simulink model "sim_all"  (R2020a)
settings: Solver=VariableStepAuto  StartTime=0.0  StopTime=2000  RelTol=1e-3
values from neighbouring files (symbols this model uses):
  a1 = rho * D^4 * alpha1    (= 0.000388302366464)    [data_current.m]
  a2 = -rho * D^3 * alpha2 * (1 - omega)    (= 0.0037030698432)    [data_current.m]
  alpha1 = 0.0113    [data_current.m]
  alpha2 = -0.0091    [data_current.m]
  cornerA = [43.781381 ... (first row only)    [missionC.m]
  cornerB = [43.780975 ... (first row only)    [missionC.m]
  cornerC = [43.780189 ... (first row only)    [missionC.m]
  cornerD = [43.780602 ... (first row only)    [missionC.m]
  ctrl_clockwise = false    [controller.m]
  ctrl_int_bound_or = 0.1    [controller.m]
  ctrl_int_bound_pos = 1    [controller.m]
  ctrl_k_or = 1    [controller.m]
  ctrl_k_pos = 1/3    (= 0.333333333333)    [controller.m]
  ctrl_Ki_vel = 100    [controller.m]
  ctrl_Kp_v_pos = 200    [controller.m]
  ctrl_Kp_vel = 200    [controller.m]
  ctrl_TAM = [  1     1           0           0               0       0;               0     0           1           1               0       0;               0     0           0           0               1       1;               0     0  -(ctrl_r+ctrl_dc)  ctrl_r+ctrl_dc    0       0;               0     0           0           0            -ctrl_r    ctrl_r;           -ctrl_r ctrl_r        0           0       ...(+19 chars)    [controller.m]
  ctrl_Ts = 0.1    [controller.m]
  ctrl_va_uncontrolled = 0.15    [controller.m]
  ctrl_vel_uncontrolled = 0.5    [controller.m]
  D = 0.076    [data_current.m]
  dead_zone_limit = 31.5    [data_current.m]
  depth = 5    [missionC.m]
  distanceFromWall = 8    [missionC.m]
  initInspectedSide = 2    [missionC.m]
  initPoint = [ 43.780796 ... (first row only)    [missionC.m]
  mod_A = pi*mod_R*mod_R    [model.m]
  mod_Cd_F = 0.45    [model.m]
  mod_Cd_M = 0.4    [model.m]
  mod_eta_init = [mod_xNorth; mod_yEast; -mod_zDown; 0; 0; 0]    [model.m]
  mod_g = 9.81    [model.m]
  mod_h0 = 0    [model.m]
  mod_Ixx = mod_Io(1,1)    [model.m]
  mod_Iyy = mod_Io(2,2)    [model.m]
  mod_Izz = mod_Io(3,3)    [model.m]
  mod_Kp_dot = 0    [model.m]
  mod_lat0 = 43.780189    [model.m]
  mod_lon0 = 11.282698    [model.m]
  mod_m = 100    [model.m]
  mod_Mq_dot = mod_Kp_dot    (= 0)    [model.m]
  mod_ni_init = [0; 0; 0; 0; 0; 0]    [model.m]
  mod_Nr_dot = mod_Kp_dot    (= 0)    [model.m]
  mod_p1 = [0; mod_R; 0]    [model.m]
  mod_p2 = [0; -mod_R; 0]    [model.m]
  mod_p3 = [0; 0; (mod_R + mod_z_cm)]    [model.m]
  mod_p4 = [0; 0; -(mod_R + mod_z_cm)]    [model.m]
  mod_p5 = [mod_R; 0; 0]    [model.m]
  mod_p6 = [-mod_R; 0; 0]    [model.m]
  mod_R = ((3*mod_Vol)/(4*pi))^(1/3)    [model.m]
  mod_Rm = (4*mod_R)/(3*pi)    [model.m]
  mod_t1 = [1; 0; 0]    [model.m]
  mod_t2 = [1; 0; 0]    [model.m]
  mod_t3 = [0; 1; 0]    [model.m]
  mod_t4 = [0; 1; 0]    [model.m]
  mod_t5 = [0; 0; 1]    [model.m]
  mod_t6 = [0; 0; 1]    [model.m]
  mod_W = mod_m*mod_g    (= 981)    [model.m]
  mod_Xu_dot = (2/3)*mod_rho_AUV*pi*(mod_R^3)    [model.m]
  mod_Yv_dot = mod_Xu_dot    [model.m]
  mod_z_cm = mod_r_cm(3)    [model.m]
  mod_Zw_dot = mod_Xu_dot    [model.m]
  n_max = 340    [data_current.m]
  nav_DT = 0.1    [navigation.m]
  nav_filter = -1    [data_analysis_simulation_total.m]    (also in navigation.m)
  nav_giro = 2    [navigation.m]
  nav_h0 = 0    [navigation.m]
  nav_lat0 = cornerC(1)    [navigation.m]
  nav_lon0 = cornerC(2)    [navigation.m]
  nav_plane_AB = coefficient_plane(nav_A,nav_B)    [navigation.m]
  nav_plane_BC = coefficient_plane(nav_B,nav_C)    [navigation.m]
  nav_plane_CD = coefficient_plane(nav_C,nav_D)    [navigation.m]
  nav_plane_DA = coefficient_plane(nav_D,nav_A)    [navigation.m]
  nav_resampling = 10000    [navigation.m]
  omega = 0.1    [data_current.m]
  relativeDirection = 30    [missionC.m]
  res_enable_n_eff = 1    [navigation.m]
  rho = 1030    [data_current.m]
  sens_distCM = 0.267    [sensors.m]
  sens_Sample_time_AHRS = 0.1    [sensors.m]
  sens_Sample_time_depth = 0.1    [sensors.m]
  sens_Sample_time_dvl = 0.2    [sensors.m]
  sens_Sample_time_GPS = 1    [sensors.m]
  sens_Sample_time_GYRO = 0.1    [sensors.m]
  sens_Sample_time_sonar = 0.5    [sensors.m]
  sens_threshold = 0.485    [sensors.m]
  sens_Variance_AHRS_pitch = (0.0087)^2    (= 7.569e-05)    [sensors.m]
  sens_Variance_AHRS_roll = (0.0087)^2    (= 7.569e-05)    [sensors.m]
  sens_Variance_AHRS_yaw = (0.0017)^2    (= 2.89e-06)    [sensors.m]
  sens_Variance_depth1 = (0.2)^2    (= 0.04)    [sensors.m]
  sens_Variance_depth2 = (0.4)^2    (= 0.16)    [sensors.m]
  sens_Variance_DVL = (speed*0.03)^2    [sensors.m]
  sens_Variance_GPS = 3    [sensors.m]
  sens_Variance_GYRO = 2.5133e-06    [sensors.m]
  sens_Variance_sonar = 0.05    [sensors.m]
  soglia_or = [0.1, 0.1, 0.1]    [mission.m]
  soglia_orp = 0.1    [mission.m]
  soglia_parete = 0.5    [mission.m]
  soglia_parete_frenata = 0.5    [mission.m]
  soglia_pos = [0.00001, 0.00001, 0.5]    [mission.m]
  soglia_SOS_collisione = 2    [mission.m]
  soglia_SOS_or = [0.25, 0.25, 0.25]    [mission.m]
  soglia_SOS_orp = 0.25    [mission.m]
  soglia_SOS_parete = 1    [mission.m]
  soglia_SOS_pos = [0.00005, 0.00005, 1]    [mission.m]
  soglia_SOS_pos_ris = 2    [mission.m]
  soglia_SOS_vel = 0.2    [mission.m]
  SOS = 0    [mission.m]
  speed = 0.4    [missionC.m]
  stato = 100    [mission.m]
  timer = 40*2    (= 80)    [mission.m]
  Ts_supervisor = 0.1    [mission.m]
undefined symbols (not defined in the file or in its folder): DiscIntNeverNeededParam, nav_A, nav_B, nav_C, nav_D
libraries: simulink x8, cstblocks x6, simulink_extras x1
(part 3 of 8)

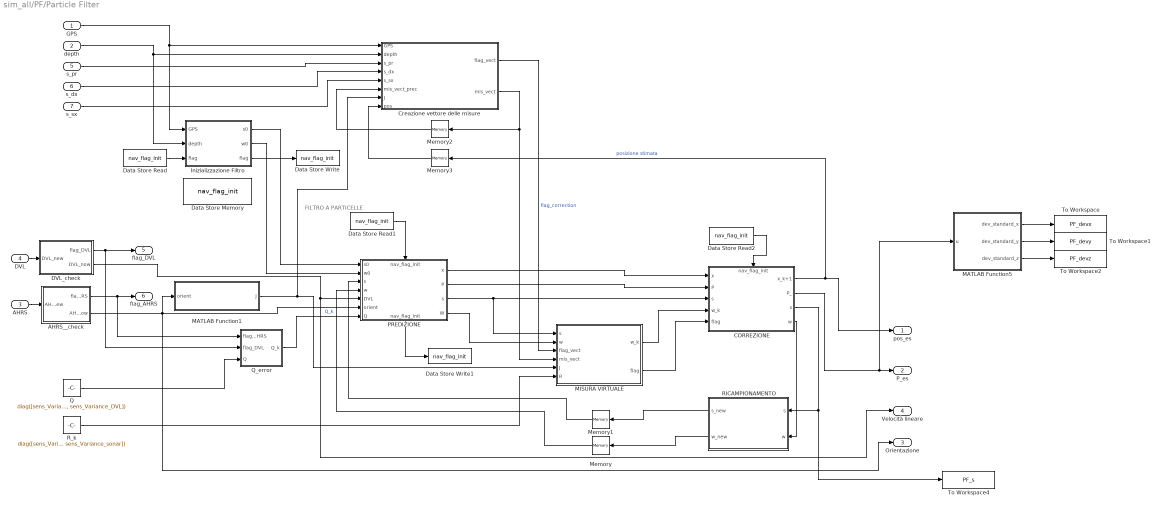
== system sim_all/PF/Particle Filter ==
  note: FILTRO A PARTICELLE
  GPS : Inport
  depth : Inport  Port=2
  AHRS : Inport  Port=3
  DVL : Inport  Port=4
  s_pr : Inport  Port=5
  s_dx : Inport  Port=6
  s_sx : Inport  Port=7
  AHRS__check : Subsystem
  CORREZIONE : Subsystem
      settings: PortSchema="{\"entries\":[{\"content\":{\"sides\":[{\"content\":{\"connectorIds\":[\"In1\",\"In2\",\"In3\",\"In4\",\"In5\"]},\"type\":\"ConnectorPlacement.EquallySpacedRectSide\",\"uuid\":\"067d30f7-0887-4b4f-a6ee-617ba2d59620\"},{\"content\":{\"connectorIds\":[\"Out1\",\"Out2\",\"Out3\",\"Out4\"],\"side\":\"RIGHT\"},\"type\":\"ConnectorPlacement.EquallySpacedRectSide\",\"uuid\":\"6eaec154-fa9b-4277-964e-a31b5cab1928\"},{\"content\":{\"connectorIds\":[\"In6\"],\"side\":\"TOP\"},\"type\":\"ConnectorPlacement.EquallySpacedRectSide\",\"uuid\":\"eb829d42-6933-4b20-85d8-52dfe5077273\"}]},\"type\":\"ConnectorPlacement.EquallySpacedConnector\",\"uuid\":\"d9ec3b67-6d70-427e-aad1-a2dcdcd4b00e\"}],\"packageUris\":[\"http://schema.mathworks.com/mf0/Connector/19700101\"],\"version\":\"1.0\"}"
  Creazione vettore delle misure : MATLAB Function  TreatAsAtomicUnit=on  SystemSampleTime=nav_DT
  DVL_check : Subsystem
  Data Store Memory : DataStoreMemory  DataStoreName=nav_flag_init  ShowAdditionalParam=off
  Data Store Read : DataStoreRead  DataStoreName=nav_flag_init  DataStoreElements=nav_flag_init
  Data Store Read1 : DataStoreRead  DataStoreName=nav_flag_init  DataStoreElements=nav_flag_init
  Data Store Read2 : DataStoreRead  DataStoreName=nav_flag_init  DataStoreElements=nav_flag_init
  Data Store Write : DataStoreWrite  DataStoreName=nav_flag_init  DataStoreElements=nav_flag_init
  Data Store Write1 : DataStoreWrite  DataStoreName=nav_flag_init  DataStoreElements=nav_flag_init
  Inizializzazione Filtro : MATLAB Function  TreatAsAtomicUnit=on  SystemSampleTime=nav_DT
  MATLAB Function1 : MATLAB Function  TreatAsAtomicUnit=on
  MATLAB Function5 : MATLAB Function  TreatAsAtomicUnit=on
  MISURA VIRTUALE : Subsystem
  Memory{,1..3} (4 alike) : Memory
  PREDIZIONE : Subsystem
      settings: PortSchema="{\"entries\":[{\"content\":{\"sides\":[{\"content\":{\"connectorIds\":[\"In1\",\"In2\",\"In3\",\"In4\",\"In5\",\"In6\",\"In7\"]},\"type\":\"ConnectorPlacement.EquallySpacedRectSide\",\"uuid\":\"d45a5da5-05d0-4cdd-84b6-a248ae6e7ceb\"},{\"content\":{\"connectorIds\":[\"Out1\",\"Out2\",\"Out3\",\"Out4\"],\"side\":\"RIGHT\"},\"type\":\"ConnectorPlacement.EquallySpacedRectSide\",\"uuid\":\"47480e48-a9e6-47c5-bf02-88857c9c5826\"},{\"content\":{\"connectorIds\":[\"In8\"],\"side\":\"TOP\"},\"type\":\"ConnectorPlacement.EquallySpacedRectSide\",\"uuid\":\"fce086aa-2512-4880-8bcd-6ad591a282b2\"},{\"content\":{\"connectorIds\":[\"Out5\"],\"side\":\"BOTTOM\"},\"type\":\"ConnectorPlacement.EquallySpacedRectSide\",\"uuid\":\"b6d1202f-9ea1-4bf5-aa1c-3bdf29b80993\"}]},\"type\":\"ConnectorPlacement.EquallySpacedConnector\",\"uuid\":\"773da45d-9f7f-4876-9289-a755558658b5\"}],\"packageUris\":[\"http://schema.mathworks.com/mf0/Connector/19700101\"],\"version\":\"1.0\"}"
  Q : Constant  Value=diag([sens_Variance_AHRS_roll, sens_Variance_AHRS_pitch, sens_Variance_AHRS_yaw, sens_Variance_DVL, sens_Variance_DVL, sens_Variance_DVL])  VectorParams1D=off
  Q_error : Subsystem
  RICAMPIONAMENTO : Subsystem
  R_k : Constant  Value=diag([sens_Variance_GPS, sens_Variance_GPS, sens_Variance_depth1, sens_Variance_sonar, sens_Variance_sonar, sens_Variance_sonar])  VectorParams1D=off
  To Workspace : ToWorkspace  VariableName=PF_devx  SaveFormat=Timeseries  SampleTime=0.1
      settings: Decimation=10
  To Workspace1 : ToWorkspace  VariableName=PF_devy  SaveFormat=Timeseries  SampleTime=0.1
      settings: Decimation=10
  To Workspace2 : ToWorkspace  VariableName=PF_devz  SaveFormat=Timeseries  SampleTime=0.1
      settings: Decimation=10
  To Workspace4 : ToWorkspace  VariableName=PF_s  SaveFormat=Timeseries  SampleTime=0.1
      settings: Decimation=10
  pos_es : Outport  PortDimensions=3
  P_es : Outport  Port=2
  Orientazione : Outport  Port=3
  Velocità lineare : Outport  Port=4
  flag_DVL : Outport  Port=5
  flag_AHRS : Outport  Port=6
  wires:
  Memory/1 -> PREDIZIONE/4(w)
  CORREZIONE/2(P_) -> MATLAB Function5/1(u), P_es/1
  Memory1/1 -> PREDIZIONE/3("s ")
  GPS/1 -> Inizializzazione Filtro/1(GPS), Creazione vettore delle misure/1(GPS)
  depth/1 -> Inizializzazione Filtro/2(depth), Creazione vettore delle misure/2(depth)
  s_pr/1 -> Creazione vettore delle misure/3(s_pr)
  Creazione vettore delle misure/2(mis_vect) -> MISURA VIRTUALE/4(mis_vect), Memory2/1
  Memory2/1 -> Creazione vettore delle misure/6(mis_vect_prec)
  s_dx/1 -> Creazione vettore delle misure/4(s_dx)
  s_sx/1 -> Creazione vettore delle misure/5(s_sx)
  Inizializzazione Filtro/2(w0) -> PREDIZIONE/2(w0)
  Inizializzazione Filtro/1(s0) -> PREDIZIONE/1(s0)
  MATLAB Function1/1(J) -> Creazione vettore delle misure/7(J), MISURA VIRTUALE/5(J)
  Data Store Read/1 -> Inizializzazione Filtro/3("flag ")
  Inizializzazione Filtro/3(flag) -> Data Store Write/1
  Data Store Read1/1 -> PREDIZIONE/8("nav_flag_init ")
  Data Store Read2/1 -> CORREZIONE/6(nav_flag_init)
  PREDIZIONE/5(nav_flag_init) -> Data Store Write1/1
  CORREZIONE/1(x_k+1) -> pos_es/1, Memory3/1  "posizione stimata"
  Memory3/1 -> Creazione vettore delle misure/8(pos)
  AHRS__check/2(AHRS_now) -> PREDIZIONE/6(orient), MATLAB Function1/1(orient), Orientazione/1
  DVL_check/2(DVL_now) -> PREDIZIONE/5(DVL), Velocità lineare/1
  DVL/1 -> DVL_check/1(DVL_new)
  AHRS/1 -> AHRS__check/1(AHRS_new)
  DVL_check/1(flag_DVL) -> flag_DVL/1, Q_error/2(flag_DVL)
  AHRS__check/1(flag_AHRS) -> flag_AHRS/1, Q_error/1(flag_AHRS)
  Q/1 -> Q_error/3(Q)
  Q_error/1(Q_k) -> PREDIZIONE/7(Q)  "Q_k"
  MISURA VIRTUALE/2(flag) -> CORREZIONE/5(flag)
  MISURA VIRTUALE/1(w_k) -> CORREZIONE/4(w_k)
  RICAMPIONAMENTO/1(s_new) -> Memory1/1
  RICAMPIONAMENTO/2(w_new) -> Memory/1
  CORREZIONE/3("s ") -> To Workspace4/1, RICAMPIONAMENTO/1("s ")
  CORREZIONE/4(w) -> RICAMPIONAMENTO/2(w)
  R_k/1 -> MISURA VIRTUALE/6(R)
  Creazione vettore delle misure/1(flag_vect) -> MISURA VIRTUALE/3(flag_vect)  "flag_correction"
  PREDIZIONE/1(x) -> CORREZIONE/1(x)
  PREDIZIONE/2(P) -> CORREZIONE/2(P)
  PREDIZIONE/3(s) -> MISURA VIRTUALE/1(s), CORREZIONE/3(s)
  MATLAB Function5/1(dev_standard_x) -> To Workspace/1
  MATLAB Function5/3(dev_standard_z) -> To Workspace2/1
  MATLAB Function5/2(dev_standard_y) -> To Workspace1/1
  PREDIZIONE/4(W) -> MISURA VIRTUALE/2(w)

== system sim_all/PF/SOS_flag_generator ==
  P_es : Inport
  AHRS : Inport  Port=2
  DVL : Inport  Port=3
  Gyro : Inport  Port=4
  MATLAB Function : MATLAB Function  TreatAsAtomicUnit=on  SystemSampleTime=nav_DT
  Memory : Memory
  nav_SOS : Outport
  tag scope: nav_contatore=global
  wires:
  MATLAB Function/1(SOS) -> nav_SOS/1
  AHRS/1 -> MATLAB Function/3(AHRS)
  DVL/1 -> MATLAB Function/2(DVL)
  P_es/1 -> MATLAB Function/1(P_es)
  [nav_contatore] -> Memory/1
  MATLAB Function/2(contatore) -> [nav_contatore]
  Gyro/1 -> MATLAB Function/4(gyro)
  Memory/1 -> MATLAB Function/5("contatore ")

== system sim_all/Sensors/BLOCCO AHRS1 ==
  note: R  [rad]
      | P  [rad]
  note: Y [rad]
  orient_real : Inport  SampleTime=sens_Sample_time_AHRS
  orient_real1 : Inport  Port=2  SampleTime=sens_Sample_time_AHRS
  orient_real2 : Inport  Port=3  SampleTime=sens_Sample_time_AHRS
  Mux2 : Mux  Inputs=2
  Quantizer : Quantizer  QuantizationInterval=sens_Resolution_AHRS  LinearizeAsGain=off
  Quantizer1 : Quantizer  QuantizationInterval=sens_Resolution_AHRS  LinearizeAsGain=off
  Quantizer2 : Quantizer  QuantizationInterval=sens_Resolution_AHRS  LinearizeAsGain=off
  Random Number : RandomNumber  Variance=sens_Variance_AHRS_roll  Seed=5678  SampleTime=sens_Sample_time_AHRS
  Random Number1 : RandomNumber  Variance=sens_Variance_AHRS_pitch  Seed=4562  SampleTime=sens_Sample_time_AHRS
  Random Number2 : RandomNumber  Variance=sens_Variance_AHRS_yaw  Seed=1258  SampleTime=sens_Sample_time_AHRS
  Sum1 : Sum  Inputs=|++
  Sum2 : Sum  Inputs=++|
  Sum6 : Sum  Inputs=|++
  R-P NED : Outport
  Y NED : Outport  Port=2
  wires:
  orient_real2/1 -> Sum6/1
  orient_real/1 -> Sum2/2
  Sum6/1 -> Quantizer2/1
  Mux2/1 -> R-P NED/1
  Sum2/1 -> Quantizer/1
  orient_real1/1 -> Sum1/1
  Random Number1/1 -> Sum1/2
  Sum1/1 -> Quantizer1/1
  Random Number/1 -> Sum2/1
  Random Number2/1 -> Sum6/2
  Quantizer/1 -> Mux2/1
  Quantizer1/1 -> Mux2/2
  Quantizer2/1 -> Y NED/1

== system sim_all/Sensors/BLOCCO DVL1 ==
  "DVL vx " : Inport  SampleTime=sens_Sample_time_dvl
  DVL vy : Inport  Port=2  SampleTime=sens_Sample_time_dvl
  DVL vz : Inport  Port=3  SampleTime=sens_Sample_time_dvl
  " WNoise DVL x " : RandomNumber  Variance=sens_Variance_DVL  Seed=1234  SampleTime=sens_Sample_time_dvl
  Quantizer : Quantizer  QuantizationInterval=sens_Resolution_dvl  LinearizeAsGain=off
  Quantizer1 : Quantizer  QuantizationInterval=sens_Resolution_dvl  LinearizeAsGain=off
  Quantizer2 : Quantizer  QuantizationInterval=sens_Resolution_dvl  LinearizeAsGain=off
  Sum1 : Sum  Inputs=|++
  Sum2 : Sum  Inputs=|++
  Sum3 : Sum  Inputs=|++
  WNoise DVL y : RandomNumber  Variance=sens_Variance_DVL  Seed=1235  SampleTime=sens_Sample_time_dvl
  WNoise DVL z : RandomNumber  Variance=sens_Variance_DVL  Seed=1237  SampleTime=sens_Sample_time_dvl
  DVL vx BODY : Outport
  DVL vy BODY : Outport  Port=2
  DVL vz BODY : Outport  Port=3
  wires:
  " WNoise DVL x "/1 -> Sum2/2
  Sum2/1 -> Quantizer/1
  WNoise DVL y/1 -> Sum1/2
  Sum1/1 -> Quantizer1/1
  WNoise DVL z/1 -> Sum3/2
  Sum3/1 -> Quantizer2/1
  "DVL vx "/1 -> Sum2/1
  DVL vy/1 -> Sum1/1
  DVL vz/1 -> Sum3/1
  Quantizer/1 -> DVL vx BODY/1
  Quantizer1/1 -> DVL vy BODY/1
  Quantizer2/1 -> DVL vz BODY/1

== system sim_all/Sensors/BLOCCO GPS1 ==
  note: Controllo per antenna
  "LAT " : Inport  SampleTime=sens_Sample_time_GPS
  "LON " : Inport  Port=2  SampleTime=sens_Sample_time_GPS
  DEP : Inport  Port=3  SampleTime=sens_Sample_time_GPS
  Compare To Constant : simulink/Logic and Bit Operations/Compare To Constant  relop=<  const=sens_threshold  OutDataTypeStr=uint8
  Quantizer : Quantizer  QuantizationInterval=sens_Resolution_GPS
  Quantizer1 : Quantizer  QuantizationInterval=sens_Resolution_GPS  LinearizeAsGain=off
  Sum2 : Sum  Inputs=++|
  Sum3 : Sum  Inputs=|++
  WN LAT : RandomNumber  Variance=sens_Variance_GPS  Seed=8765  SampleTime=sens_Sample_time_GPS
  WN LON : RandomNumber  Variance=sens_Variance_GPS  Seed=9876  SampleTime=sens_Sample_time_GPS
  "GPS LAT " : Outport
  "GPS LON " : Outport  Port=2
  FLAG : Outport  Port=3
  wires:
  Sum3/1 -> Quantizer/1
  "LON "/1 -> Sum3/1
  WN LON/1 -> Sum3/2
  Sum2/1 -> Quantizer1/1
  Compare To Constant/1 -> FLAG/1
  DEP/1 -> Compare To Constant/1
  WN LAT/1 -> Sum2/1
  "LAT "/1 -> Sum2/2
  Quantizer1/1 -> "GPS LAT "/1
  Quantizer/1 -> "GPS LON "/1

== system sim_all/Sensors/BLOCCO GYRO1 ==
  angvel_rea1l : Inport  SampleTime=sens_Sample_time_GYRO
  angvel_real2 : Inport  Port=2  SampleTime=sens_Sample_time_GYRO
  angvel_real3 : Inport  Port=3  SampleTime=sens_Sample_time_GYRO
  Clock1 : Clock
  Quantizer : Quantizer  QuantizationInterval=sens_Resolution_GYRO  LinearizeAsGain=off
  Quantizer1 : Quantizer  QuantizationInterval=sens_Resolution_GYRO  LinearizeAsGain=off
  Quantizer2 : Quantizer  QuantizationInterval=sens_Resolution_GYRO  LinearizeAsGain=off
  Subsystem : Subsystem
  Sum1 : Sum  Inputs=+++
  Sum2 : Sum  Inputs=+++
  Sum5 : Sum  Inputs=+++
  WN Gyro P : RandomNumber  Variance=sens_Variance_GYRO  Seed=2347  SampleTime=sens_Sample_time_GYRO
  WN Gyro R : RandomNumber  Variance=sens_Variance_GYRO  Seed=2346  SampleTime=sens_Sample_time_GYRO
  WN Gyro Y : RandomNumber  Variance=sens_Variance_GYRO  Seed=2348  SampleTime=sens_Sample_time_GYRO
  Gyro R BODY : Outport
  Gyro P BODY : Outport  Port=2
  Gyro Y BODY : Outport  Port=3
  wires:
  Sum5/1 -> Quantizer/1
  Sum1/1 -> Quantizer1/1
  Sum2/1 -> Quantizer2/1
  Quantizer/1 -> Gyro R BODY/1
  Quantizer1/1 -> Gyro P BODY/1
  Quantizer2/1 -> Gyro Y BODY/1
  angvel_rea1l/1 -> Sum5/2
  angvel_real2/1 -> Sum1/2
  WN Gyro P/1 -> Sum1/3
  angvel_real3/1 -> Sum2/2
  WN Gyro Y/1 -> Sum2/3
  Clock1/1 -> Subsystem/1(t)
  Subsystem/1(Bias_G) -> Sum2/1, Sum1/1, Sum5/1
  WN Gyro R/1 -> Sum5/3

== system sim_all/Sensors/BLOCCO PROF.1 ==
  note: [m]
  DEP : Inport  SampleTime=sens_Sample_time_depth
  Compare To Constant1 : simulink/Logic and Bit Operations/Compare To Constant  relop=<  const=50  OutDataTypeStr=boolean
  Quantizer : Quantizer  QuantizationInterval=sens_Resolution_depth  LinearizeAsGain=off
  Sum3 : Sum  Inputs=++|
  Switch : Switch  Criteria=u2 > Threshold
  "WN Prof. h< 50 " : RandomNumber  Variance=sens_Variance_depth1  Seed=6543  SampleTime=sens_Sample_time_depth
  WN Prof. h>50 : RandomNumber  Variance=sens_Variance_depth2  Seed=3210  SampleTime=sens_Sample_time_depth
  Profondimetro : Outport
  wires:
  DEP/1 -> Sum3/2, Compare To Constant1/1
  Compare To Constant1/1 -> Switch/2
  "WN Prof. h< 50 "/1 -> Switch/1
  WN Prof. h>50/1 -> Switch/3
  Switch/1 -> Sum3/1
  Sum3/1 -> Quantizer/1
  Quantizer/1 -> Profondimetro/1

== system sim_all/Sensors/Environment and Sensors Model3 ==
  LAT-LON : Inport  SampleTime=sens_Sample_time_sonar
  Environment : Inport  Port=2  SampleTime=sens_Sample_time_sonar
  AHRS Roll : Inport  Port=3  SampleTime=sens_Sample_time_sonar
  AHRS Pitch : Inport  Port=4  SampleTime=sens_Sample_time_sonar
  AHRS Yaw : Inport  Port=5  SampleTime=sens_Sample_time_sonar
  " WN Sonar DX " : RandomNumber  Variance=sens_Variance_sonar  Seed=4325  SampleTime=sens_Sample_time_sonar
  Constant : Constant  Value=sens_distCM
  Demux3 : Demux  Outputs=5
  MATLAB Function1 : MATLAB Function  TreatAsAtomicUnit=on
  Quantizer : Quantizer  QuantizationInterval=sens_Resolution_sonar  LinearizeAsGain=off
  Sum1 : Sum  Inputs=|+-
  Sum2 : Sum  Inputs=|++
  Sonar DX : Outport
  wires:
  MATLAB Function1/1(dist) -> Sum1/1
  Sum1/1 -> Sum2/1
  Constant/1 -> Sum1/2
  Environment/1 -> Demux3/1
  Quantizer/1 -> Sonar DX/1
  Demux3/4 -> MATLAB Function1/5(plane_DA)
  Demux3/2 -> MATLAB Function1/3(plane_BC)
  Sum2/1 -> Quantizer/1
  Demux3/3 -> MATLAB Function1/4(plane_CD)
  AHRS Pitch/1 -> MATLAB Function1/8(Pitch)
  Demux3/1 -> MATLAB Function1/2(plane_AB)
  AHRS Roll/1 -> MATLAB Function1/7(Roll)
  AHRS Yaw/1 -> MATLAB Function1/9(Yaw)
  " WN Sonar DX "/1 -> Sum2/2
  LAT-LON/1 -> MATLAB Function1/1(pos)
  Demux3/5 -> MATLAB Function1/6(plane_W)

== system sim_all/Sensors/Environment and Sensors Model4 ==
  LAT-LON : Inport  SampleTime=sens_Sample_time_sonar
  Environment : Inport  Port=2  SampleTime=sens_Sample_time_sonar
  AHRS Roll : Inport  Port=3  SampleTime=sens_Sample_time_sonar
  AHRS Pitch : Inport  Port=4  SampleTime=sens_Sample_time_sonar
  AHRS Yaw : Inport  Port=5  SampleTime=sens_Sample_time_sonar
  " WN Sonar SX " : RandomNumber  Variance=sens_Variance_sonar  Seed=4321  SampleTime=sens_Sample_time_sonar
  Constant : Constant  Value=sens_distCM
  Demux3 : Demux  Outputs=5
  MATLAB Function1 : MATLAB Function  TreatAsAtomicUnit=on
  Quantizer : Quantizer  QuantizationInterval=sens_Resolution_sonar  LinearizeAsGain=off
  Sum1 : Sum  Inputs=|+-
  Sum2 : Sum  Inputs=|++
  Sonar SX : Outport
  wires:
  MATLAB Function1/1(dist) -> Sum1/1
  Sum1/1 -> Sum2/1
  Constant/1 -> Sum1/2
  Environment/1 -> Demux3/1
  Quantizer/1 -> Sonar SX/1
  Demux3/4 -> MATLAB Function1/5(plane_DA)
  Demux3/2 -> MATLAB Function1/3(plane_BC)
  Sum2/1 -> Quantizer/1
  Demux3/3 -> MATLAB Function1/4(plane_CD)
  AHRS Pitch/1 -> MATLAB Function1/8(Pitch)
  Demux3/1 -> MATLAB Function1/2(plane_AB)
  AHRS Roll/1 -> MATLAB Function1/7(Roll)
  AHRS Yaw/1 -> MATLAB Function1/9(Yaw)
  " WN Sonar SX "/1 -> Sum2/2
  LAT-LON/1 -> MATLAB Function1/1(pos)
  Demux3/5 -> MATLAB Function1/6(plane_W)

== system sim_all/Sensors/Environment and Sensors Model6 ==
  LAT-LON : Inport  SampleTime=sens_Sample_time_sonar
  Environment : Inport  Port=2  SampleTime=sens_Sample_time_sonar
  AHRS Roll : Inport  Port=3  SampleTime=sens_Sample_time_sonar
  AHRS Pitch : Inport  Port=4  SampleTime=sens_Sample_time_sonar
  AHRS Yaw : Inport  Port=5  SampleTime=sens_Sample_time_sonar
  " WN Sonar Prua " : RandomNumber  Variance=sens_Variance_sonar  Seed=1234  SampleTime=sens_Sample_time_sonar
  Constant : Constant  Value=sens_distCM
  Demux3 : Demux  Outputs=5
  MATLAB Function1 : MATLAB Function  TreatAsAtomicUnit=on
  Quantizer : Quantizer  QuantizationInterval=sens_Resolution_sonar  LinearizeAsGain=off
  Sum1 : Sum  Inputs=|+-
  Sum2 : Sum  Inputs=|++
  Sonar Prua : Outport
  wires:
  Demux3/3 -> MATLAB Function1/4(plane_CD)
  " WN Sonar Prua "/1 -> Sum2/2
  LAT-LON/1 -> MATLAB Function1/1(pos)
  Demux3/1 -> MATLAB Function1/2(plane_AB)
  Demux3/4 -> MATLAB Function1/5(plane_DA)
  Sum2/1 -> Quantizer/1
  Demux3/2 -> MATLAB Function1/3(plane_BC)
  Quantizer/1 -> Sonar Prua/1
  Environment/1 -> Demux3/1
  AHRS Roll/1 -> MATLAB Function1/7(Roll)
  AHRS Pitch/1 -> MATLAB Function1/8(Pitch)
  AHRS Yaw/1 -> MATLAB Function1/9(Yaw)
  MATLAB Function1/1(dist) -> Sum1/1
  Sum1/1 -> Sum2/1
  Constant/1 -> Sum1/2
  Demux3/5 -> MATLAB Function1/6(plane_W)

== system sim_all/Controller_mk4_v3/C_or/C_va_X_td ==
  err_va : Inport
  Reset : ResetPort  DisableCoverage=on
  LTI System : cstblocks/LTI System  sys=ctrl_Cva_td3  IC=[]
  tau : Outport
  wires:
  err_va/1 -> LTI System/1
  LTI System/1 -> tau/1

== system sim_all/Controller_mk4_v3/C_or/C_va_Y_td ==
  err_va : Inport
  Reset : ResetPort  DisableCoverage=on
  LTI System : cstblocks/LTI System  sys=ctrl_Cva_td3  IC=[]
  tau : Outport
  wires:
  LTI System/1 -> tau/1
  err_va/1 -> LTI System/1

== system sim_all/Controller_mk4_v3/C_or/C_va_Z_td ==
  err_va : Inport
  Reset : ResetPort  DisableCoverage=on
  LTI System : cstblocks/LTI System  sys=ctrl_Cva_td3  IC=[]
  tau : Outport
  wires:
  err_va/1 -> LTI System/1
  LTI System/1 -> tau/1

== system sim_all/Controller_mk4_v3/C_pos/abs_integrator1 ==
  err_x : Inport
  err_y : Inport  Port=2
  err_z : Inport  Port=3
  enabler : Inport  Port=4
  Body2Ned : MATLAB Function  TreatAsAtomicUnit=on
  Demux : Demux  Outputs=3
  Discrete-Time Integrator : DiscreteIntegrator  gainval=ctrl_Ki_pos  ExternalReset=rising  SampleTime=ctrl_Ts  ICPrevOutput=DiscIntNeverNeededParam  ICPrevScaledInput=DiscIntNeverNeededParam
  Mux : Mux  Inputs=3
  Ned2Body1 : MATLAB Function  TreatAsAtomicUnit=on
  int_x : Outport
  int_y : Outport  Port=2
  int_z : Outport  Port=3
  wires:
  [Or] -> Ned2Body1/2(or), Body2Ned/2(or)
  enabler/1 -> Discrete-Time Integrator/2
  Body2Ned/1(x_n) -> Discrete-Time Integrator/1
  err_x/1 -> Mux/1
  err_y/1 -> Mux/2
  Mux/1 -> Body2Ned/1(x_b)
  Ned2Body1/1(x_b) -> Demux/1
  Demux/1 -> int_x/1
  Demux/2 -> int_y/1
  Demux/3 -> int_z/1
  err_z/1 -> Mux/3
  Discrete-Time Integrator/1 -> Ned2Body1/1(x_n)

== system sim_all/Controller_mk4_v3/C_pos/abs_integrator2 ==
  err_vx : Inport
  err_vy : Inport  Port=2
  err_vz : Inport  Port=3
  enabler : Inport  Port=4
  Body2Ned : MATLAB Function  TreatAsAtomicUnit=on
  Demux : Demux  Outputs=3
  Discrete-Time Integrator : DiscreteIntegrator  gainval=ctrl_Ki_v_pos  ExternalReset=rising  SampleTime=ctrl_Ts  ICPrevOutput=DiscIntNeverNeededParam  ICPrevScaledInput=DiscIntNeverNeededParam
  Mux : Mux  Inputs=3
  Ned2Body1 : MATLAB Function  TreatAsAtomicUnit=on
  int_vx : Outport
  int_vy : Outport  Port=2
  int_vz : Outport  Port=3
  wires:
  Demux/3 -> int_vz/1
  Demux/2 -> int_vy/1
  Demux/1 -> int_vx/1
  Ned2Body1/1(x_b) -> Demux/1
  Mux/1 -> Body2Ned/1(x_b)
  err_vy/1 -> Mux/2
  err_vx/1 -> Mux/1
  [Or] -> Body2Ned/2(or), Ned2Body1/2(or)
  err_vz/1 -> Mux/3
  Body2Ned/1(x_n) -> Discrete-Time Integrator/1
  enabler/1 -> Discrete-Time Integrator/2
  Discrete-Time Integrator/1 -> Ned2Body1/1(x_n)

== system sim_all/Controller_mk4_v3/C_vel/abs_integrator ==
  err_vx : Inport
  err_vy : Inport  Port=2
  err_vz : Inport  Port=3
  enabler : Inport  Port=4
  Body2Ned : MATLAB Function  TreatAsAtomicUnit=on
  Demux : Demux  Outputs=3
  Discrete-Time Integrator : DiscreteIntegrator  gainval=ctrl_Ki_vel  ExternalReset=rising  SampleTime=ctrl_Ts  ICPrevOutput=DiscIntNeverNeededParam  ICPrevScaledInput=DiscIntNeverNeededParam
  Mux : Mux  Inputs=3
  Ned2Body1 : MATLAB Function  TreatAsAtomicUnit=on
  int_vx : Outport
  int_vy : Outport  Port=2
  int_vz : Outport  Port=3
  wires:
  Demux/3 -> int_vz/1
  Demux/2 -> int_vy/1
  Demux/1 -> int_vx/1
  Ned2Body1/1(x_b) -> Demux/1
  Mux/1 -> Body2Ned/1(x_b)
  err_vy/1 -> Mux/2
  err_vx/1 -> Mux/1
  [Or] -> Body2Ned/2(or), Ned2Body1/2(or)
  err_vz/1 -> Mux/3
  Body2Ned/1(x_n) -> Discrete-Time Integrator/1
  enabler/1 -> Discrete-Time Integrator/2
  Discrete-Time Integrator/1 -> Ned2Body1/1(x_n)

== system sim_all/Controller_mk4_v3/signal_to_NED/Signal_d->NED ==
  Vel_d : Inport
  Dpp_d : Inport  Port=2
  Dps_d : Inport  Port=3
  Orp_d : Inport  Port=4
  Wall : Inport  Port=5
  ToNed : MATLAB Function  TreatAsAtomicUnit=on
  wall_fcn : MATLAB Function  TreatAsAtomicUnit=on
  Vel_d_ned : Outport  VectorParamsAs1DForOutWhenUnconnected=off
  Dpp_d_ned : Outport  Port=2  VectorParamsAs1DForOutWhenUnconnected=off
  Dps_d_ned : Outport  Port=3  VectorParamsAs1DForOutWhenUnconnected=off
  Orp_d_ned : Outport  Port=4  VectorParamsAs1DForOutWhenUnconnected=off
  wires:
  wall_fcn/1(wall_vect) -> ToNed/5(wall_vect)
  ToNed/3(dps_n) -> Dps_d_ned/1
  Wall/1 -> wall_fcn/1(WALL)
  Dpp_d/1 -> ToNed/2(ddp)
  ToNed/2(ddp_n) -> Dpp_d_ned/1
  ToNed/1(vel_n) -> Vel_d_ned/1
  Orp_d/1 -> ToNed/4(orp)
  ToNed/4(orp_n) -> Orp_d_ned/1
  Dps_d/1 -> ToNed/3(dps)
  Vel_d/1 -> ToNed/1(vel)
  wall_fcn/2(wall_vect2) -> ToNed/6(wall_vect2)
  [current_state] -> ToNed/7(state)

== system sim_all/Controller_mk4_v3/signal_to_NED/Signal_s->NED ==
  Dpp_s : Inport
  Dps_s : Inport  Port=2
  Wall : Inport  Port=3
  ToNed : MATLAB Function  TreatAsAtomicUnit=on
  wall_fcn1 : MATLAB Function  TreatAsAtomicUnit=on
  Dpp_s_ned : Outport  VectorParamsAs1DForOutWhenUnconnected=off
  Dps_s_ned : Outport  Port=2  VectorParamsAs1DForOutWhenUnconnected=off
  wires:
  Dpp_s/1 -> ToNed/1(ddp)
  ToNed/1(ddp_n) -> Dpp_s_ned/1
  Dps_s/1 -> ToNed/2(dps)
  ToNed/2(dps_n) -> Dps_s_ned/1
  Wall/1 -> wall_fcn1/1(WALL)
  wall_fcn1/1(wall_vect) -> ToNed/3(wall_vect)
  wall_fcn1/2(wall_vect2) -> ToNed/4(wall_vect2)

== system sim_all/EKF/Extended Kalman Filter/AHRS__check ==
  AHRS_new : Inport
  MATLAB Function4 : MATLAB Function  TreatAsAtomicUnit=on
  Memory4 : Memory
  flag_AHRS : Outport
  AHRS_now : Outport  Port=2
  wires:
  AHRS_new/1 -> MATLAB Function4/1(AHRS_new)
  Memory4/1 -> MATLAB Function4/2(AHRS_old)
  MATLAB Function4/1(flag_AHRS) -> flag_AHRS/1
  MATLAB Function4/2(AHRS_now) -> Memory4/1, AHRS_now/1

== system sim_all/EKF/Extended Kalman Filter/CORREZIONE ==
  x_k|k-1 : Inport
  P_k|k-1 : Inport  Port=2
  e : Inport  Port=3
  H : Inport  Port=4
  R : Inport  Port=5
  nav_flag_init : Inport  Port=6
  MATLAB Function : MATLAB Function  TreatAsAtomicUnit=on  SystemSampleTime=nav_DT
  x_k|k : Outport
  P_k|k : Outport  Port=2
  wires:
  x_k|k-1/1 -> MATLAB Function/1(x_k_k_1)
  P_k|k-1/1 -> MATLAB Function/2(P_k_k_1)
  e/1 -> MATLAB Function/3(e)
  H/1 -> MATLAB Function/4(H)
  MATLAB Function/1(x_k) -> x_k|k/1
  MATLAB Function/2(P_k) -> P_k|k/1
  nav_flag_init/1 -> MATLAB Function/6(nav_flag_init)
  R/1 -> MATLAB Function/5(R_k)

== system sim_all/EKF/Extended Kalman Filter/DVL_check ==
  DVL_new : Inport
  MATLAB Function4 : MATLAB Function  TreatAsAtomicUnit=on
  Memory4 : Memory
  flag_DVL : Outport
  DVL_now : Outport  Port=2
  wires:
  DVL_new/1 -> MATLAB Function4/1(DVL_new)
  Memory4/1 -> MATLAB Function4/2(DVL_old)
  MATLAB Function4/1(flag_DVL) -> flag_DVL/1
  MATLAB Function4/2(DVL_now) -> Memory4/1, DVL_now/1

== system sim_all/EKF/Extended Kalman Filter/MISURA VIRTUALE ==
  x_k|k-1 : Inport
  flag_vect : Inport  Port=2
  mis_vect : Inport  Port=3
  J : Inport  Port=4
  MATLAB Function : MATLAB Function  TreatAsAtomicUnit=on  SystemSampleTime=nav_DT
  e : Outport
  H : Outport  Port=2
  wires:
  x_k|k-1/1 -> MATLAB Function/1(x_k_k_1)
  mis_vect/1 -> MATLAB Function/3(mis_vect)
  flag_vect/1 -> MATLAB Function/2(flag_vect)
  MATLAB Function/1(e) -> e/1
  MATLAB Function/2(H) -> H/1
  J/1 -> MATLAB Function/4(J)

== system sim_all/EKF/Extended Kalman Filter/PREDIZIONE ==
  x0 : Inport
  P0 : Inport  Port=2
  x_k-1|k-1 : Inport  Port=3
  u_k-1 : Inport  Port=4
  P_k-1|k-1 : Inport  Port=5
  J : Inport  Port=6
  L : Inport  Port=7
  Q_k-1 : Inport  Port=8
  nav_flag_init : Inport  Port=9
  Passo di Predizione : MATLAB Function  TreatAsAtomicUnit=on  SystemSampleTime=nav_DT
  x_k|k-1 : Outport
  P_k|k-1 : Outport  Port=2
  flag_init : Outport  Port=3
  wires:
  Passo di Predizione/1(x_k) -> x_k|k-1/1
  Passo di Predizione/2(P_k) -> P_k|k-1/1
  u_k-1/1 -> Passo di Predizione/4(u_k_1)
  x_k-1|k-1/1 -> Passo di Predizione/3(x_k_1)
  P_k-1|k-1/1 -> Passo di Predizione/5(P_k_1)
  J/1 -> Passo di Predizione/6(J)
  Q_k-1/1 -> Passo di Predizione/8(Q_k_1)
  P0/1 -> Passo di Predizione/2(P0)
  x0/1 -> Passo di Predizione/1(x0)
  L/1 -> Passo di Predizione/7(L)
  nav_flag_init/1 -> Passo di Predizione/9("nav_flag_init ")
  Passo di Predizione/3(nav_flag_init) -> flag_init/1

== system sim_all/EKF/Extended Kalman Filter/Q_error ==
  flag_AHRS : Inport
  flag_DVL : Inport  Port=2
  Q : Inport  Port=3
  MATLAB Function4 : MATLAB Function  TreatAsAtomicUnit=on
  Memory : Memory
  Q_k : Outport
  wires:
  MATLAB Function4/1(Q_k) -> Q_k/1, Memory/1
  flag_AHRS/1 -> MATLAB Function4/3(flag_AHRS)
  flag_DVL/1 -> MATLAB Function4/4(flag_DVL)
  Memory/1 -> MATLAB Function4/2(Q_k_1)
  Q/1 -> MATLAB Function4/1(Q)

== system sim_all/Mission_supervisor_v3/Mission_Supervisor/Completamento ==
  parete : Inport
  Pos_s : Inport  Port=2
  Vel_s : Inport  Port=3
  Dpp_s : Inport  Port=4
  Dps_s : Inport  Port=5
  Orp_s : Inport  Port=6
  Dps_fin : Inport  Port=7
  error_flag : Inport  Port=8
  giro : Inport  Port=9
  Action Port : ActionPort  ActionPortLabel=case [ 204 ]:
  Constant{,1..2,6} (4 alike) : Constant  Value=nan
  MATLAB Function : MATLAB Function  TreatAsAtomicUnit=on  SystemSampleTime=Ts_supervisor
  Mux : Mux  Inputs=6
  Mux1 : Mux  Inputs=3
  delta_current_comp : Outport
  delta_stato_comp : Outport  Port=2
  Outport : Outport  Port=3
  wires:
  MATLAB Function/1(delta_current_comp) -> delta_current_comp/1
  MATLAB Function/2(delta_stato_comp) -> delta_stato_comp/1
  parete/1 -> MATLAB Function/1(parete)
  MATLAB Function/3(Pos_d) -> Mux/1
  Mux/1 -> Outport/1
  MATLAB Function/4(Vel_d) -> Mux/3
  MATLAB Function/5(Dpp_d) -> Mux/4
  MATLAB Function/6(Orp_d) -> Mux/6
  Constant/1 -> Mux1/1
  Constant1/1 -> Mux1/2
  Constant6/1 -> Mux1/3
  Mux1/1 -> Mux/2
  Constant2/1 -> Mux/5
  Pos_s/1 -> MATLAB Function/2(Pos_s)
  Vel_s/1 -> MATLAB Function/3(Vel_s)
  Dpp_s/1 -> MATLAB Function/4(Dpp_s)
  Dps_s/1 -> MATLAB Function/5(Dps_s)
  Orp_s/1 -> MATLAB Function/6(Orp_s)
  Dps_fin/1 -> MATLAB Function/7(dps_fin)
  error_flag/1 -> MATLAB Function/8(error_flag)
  giro/1 -> MATLAB Function/9(giro)

== system sim_all/Mission_supervisor_v3/Mission_Supervisor/Fine missione ==
  current_state : Inport
  Action Port : ActionPort  ActionPortLabel=case [ 304 ]:
  Constant{1..7} (7 alike) : Constant  Value=nan
  MATLAB Function : MATLAB Function  TreatAsAtomicUnit=on  SystemSampleTime=Ts_supervisor
  Mux : Mux  Inputs=6
  Mux1 : Mux  Inputs=3
  delta_current_end : Outport
  Outport : Outport  Port=2
  wires:
  MATLAB Function/1(delta_current_end) -> delta_current_end/1
  current_state/1 -> MATLAB Function/1(stato)
  Mux/1 -> Outport/1
  Constant2/1 -> Mux/3
  Constant3/1 -> Mux/4
  Constant4/1 -> Mux/5
  Constant5/1 -> Mux/6
  Constant1/1 -> Mux1/1
  Constant6/1 -> Mux1/2
  Constant7/1 -> Mux1/3
  Mux1/1 -> Mux/1, Mux/2

== system sim_all/Mission_supervisor_v3/Mission_Supervisor/Frenata in completamento ==
  Pos_s : Inport
  Orp_s : Inport  Port=2
  Dpp_s : Inport  Port=3
  Dps_s : Inport  Port=4
  dps_fin : Inport  Port=5
  error_flag : Inport  Port=6
  Action Port : ActionPort  ActionPortLabel=case [ 205 ]:
  Constant{,1..2,6} (4 alike) : Constant  Value=nan
  MATLAB Function : MATLAB Function  TreatAsAtomicUnit=on  SystemSampleTime=Ts_supervisor
  Mux : Mux  Inputs=6
  Mux1 : Mux  Inputs=3
  delta_current_fren_comp : Outport
  delta_stato_fren_comp : Outport  Port=2
  SOS_205 : Outport  Port=3
  " " : Outport  Port=4
  wires:
  MATLAB Function/1(delta_current_fren_comp) -> delta_current_fren_comp/1
  MATLAB Function/2(delta_stato_fren_comp) -> delta_stato_fren_comp/1
  MATLAB Function/4(Pos_d) -> Mux/1
  MATLAB Function/5(Dpp_d) -> Mux/4
  MATLAB Function/6(Dps_d) -> Mux/5
  MATLAB Function/7(Orp_d) -> Mux/6
  Constant/1 -> Mux1/1
  Constant1/1 -> Mux1/2
  Constant6/1 -> Mux1/3
  Mux1/1 -> Mux/2
  Constant2/1 -> Mux/3
  Pos_s/1 -> MATLAB Function/1(Pos_s)
  Orp_s/1 -> MATLAB Function/2(Orp_s)
  Dpp_s/1 -> MATLAB Function/3(Dpp_s)
  Dps_s/1 -> MATLAB Function/4(Dps_s)
  dps_fin/1 -> MATLAB Function/5(dps_fin)
  error_flag/1 -> MATLAB Function/6(error_flag)
  MATLAB Function/3(SOS_205) -> SOS_205/1
  Mux/1 -> " "/1

== system sim_all/Mission_supervisor_v3/Mission_Supervisor/Frenata pattugliamento ==
  contatore : Inport
  Pos_s : Inport  Port=2
  Dpp_s : Inport  Port=3
  Dps_s : Inport  Port=4
  Orp_s : Inport  Port=5
  error_flag : Inport  Port=6
  Action Port : ActionPort  ActionPortLabel=case [ 202 ]:
  Constant{,1..2,6} (4 alike) : Constant  Value=nan
  MATLAB Function : MATLAB Function  TreatAsAtomicUnit=on  SystemSampleTime=Ts_supervisor
  Mux : Mux  Inputs=6
  Mux1 : Mux  Inputs=3
  delta_current_fren_patt : Outport
  delta_stato_fren_patt : Outport  Port=2
  Outport : Outport  Port=3
  wires:
  MATLAB Function/1(delta_current_fren_patt) -> delta_current_fren_patt/1
  MATLAB Function/2(delta_stato_fren_patt) -> delta_stato_fren_patt/1
  MATLAB Function/3(Pos_d) -> Mux/1
  Mux/1 -> Outport/1
  contatore/1 -> MATLAB Function/1(contatore)
  MATLAB Function/4(Dpp_d) -> Mux/4
  MATLAB Function/5(Dps_d) -> Mux/5
  MATLAB Function/6(Orp_d) -> Mux/6
  Constant/1 -> Mux1/1
  Constant1/1 -> Mux1/2
  Constant6/1 -> Mux1/3
  Mux1/1 -> Mux/2
  Constant2/1 -> Mux/3
  Pos_s/1 -> MATLAB Function/2(Pos_s)
  Dpp_s/1 -> MATLAB Function/3(Dpp_s)
  Dps_s/1 -> MATLAB Function/4(Dps_s)
  Orp_s/1 -> MATLAB Function/5(Orp_s)
  error_flag/1 -> MATLAB Function/6(error_flag)

== system sim_all/Mission_supervisor_v3/Mission_Supervisor/Immersione ==
  Pos_s : Inport
  punto_iniz_patt : Inport  Port=2
  Or_in : Inport  Port=3
  error_flag : Inport  Port=4
  Action Port : ActionPort  ActionPortLabel=case [ 103 ]:
  Constant{,1..3} (4 alike) : Constant  Value=nan
  MATLAB Function : MATLAB Function  TreatAsAtomicUnit=on  SystemSampleTime=Ts_supervisor
  Mux : Mux  Inputs=6
  delta_current_immers : Outport
  delta_stato_immers : Outport  Port=2
  Outport : Outport  Port=3
  wires:
  MATLAB Function/1(delta_current_immers) -> delta_current_immers/1
  MATLAB Function/2(delta_stato_immers) -> delta_stato_immers/1
  MATLAB Function/3(Pos_d) -> Mux/1
  Mux/1 -> Outport/1
  Constant/1 -> Mux/3
  Constant1/1 -> Mux/6
  Constant2/1 -> Mux/5
  Pos_s/1 -> MATLAB Function/1(Pos_s)
  punto_iniz_patt/1 -> MATLAB Function/2(punto_iniz_patt)
  error_flag/1 -> MATLAB Function/4(error_flag)
  MATLAB Function/4(Or_d) -> Mux/2
  Or_in/1 -> MATLAB Function/3(Or_in)
  Constant3/1 -> Mux/4

== system sim_all/Mission_supervisor_v3/Mission_Supervisor/Inizio ==
  Pos_s : Inport
  error_flag : Inport  Port=2
  Action Port : ActionPort  ActionPortLabel=case [ 100 ]:
  Constant{,1..5,7} (7 alike) : Constant  Value=nan
  Digital Clock : DigitalClock  SampleTime=0.1
  MATLAB Function : MATLAB Function  TreatAsAtomicUnit=on  SystemSampleTime=Ts_supervisor
  Mux : Mux  Inputs=6
  Mux1 : Mux  Inputs=3
  current_state : Outport
  parete_attuale : Outport  Port=2
  delta_stato : Outport  Port=3
  Outport : Outport  Port=4
  wires:
  MATLAB Function/1(current_state) -> current_state/1
  MATLAB Function/2(parete_attuale) -> parete_attuale/1
  MATLAB Function/3(stato_interno) -> delta_stato/1
  Mux/1 -> Outport/1
  Mux1/1 -> Mux/2
  Constant2/1 -> Mux/3
  Constant3/1 -> Mux/4
  Constant4/1 -> Mux/5
  Constant5/1 -> Mux/6
  Constant/1 -> Mux1/1
  Constant7/1 -> Mux1/2
  Constant1/1 -> Mux1/3
  Pos_s/1 -> MATLAB Function/1(Pos_s)
  MATLAB Function/4(Pos_d) -> Mux/1
  Digital Clock/1 -> MATLAB Function/3(attesa)
  error_flag/1 -> MATLAB Function/2(error_flag)

== system sim_all/Mission_supervisor_v3/Mission_Supervisor/Manovra ==
  contatore : Inport
  Pos_s : Inport  Port=2
  Dpp_s : Inport  Port=3
  Orp_s : Inport  Port=4
  error_flag : Inport  Port=5
  Dps_s : Inport  Port=6
  alfa : Inport  Port=7
  giro : Inport  Port=8
  parete_attuale : Inport  Port=9
  Action Port : ActionPort  ActionPortLabel=case [ 203 ]:
  Constant{,1..2,6} (4 alike) : Constant  Value=nan
  MATLAB Function : MATLAB Function  TreatAsAtomicUnit=on  SystemSampleTime=Ts_supervisor
  Mux : Mux  Inputs=6
  Mux1 : Mux  Inputs=3
  delta_current_man : Outport
  delta_stato_man : Outport  Port=2
  contatore_out : Outport  Port=3
  "  " : Outport  Port=4
  wires:
  MATLAB Function/1(delta_current_man) -> delta_current_man/1
  MATLAB Function/2(delta_stato_man) -> delta_stato_man/1
  contatore/1 -> MATLAB Function/1("contatore ")
  MATLAB Function/4(Pos_d) -> Mux/1
  Constant1/1 -> Mux/3
  MATLAB Function/5(Dpp_d) -> Mux/4
  MATLAB Function/6(Dps_d) -> Mux/5
  MATLAB Function/7(Orp_d) -> Mux/6
  Constant/1 -> Mux1/1
  Constant2/1 -> Mux1/2
  Constant6/1 -> Mux1/3
  Mux1/1 -> Mux/2
  Pos_s/1 -> MATLAB Function/2(Pos_s)
  Dpp_s/1 -> MATLAB Function/3(Dpp_s)
  Orp_s/1 -> MATLAB Function/4(Orp_s)
  error_flag/1 -> MATLAB Function/5(error_flag)
  Dps_s/1 -> MATLAB Function/6(Dps_s)
  MATLAB Function/3(contatore) -> contatore_out/1
  Mux/1 -> "  "/1
  alfa/1 -> MATLAB Function/7(alfa)
  giro/1 -> MATLAB Function/8(giro)
  parete_attuale/1 -> MATLAB Function/9(parete_attuale)

== system sim_all/Mission_supervisor_v3/Mission_Supervisor/Orientazione Iniziale ==
  Pos_s : Inport
  Or_s : Inport  Port=2
  Or_in : Inport  Port=3
  error_flag : Inport  Port=4
  Action Port : ActionPort  ActionPortLabel=case [ 101 ]:
  Constant{,1..3} (4 alike) : Constant  Value=nan
  MATLAB Function : MATLAB Function  TreatAsAtomicUnit=on  SystemSampleTime=Ts_supervisor
  Mux : Mux  Inputs=6
  delta_current_or_iniz : Outport
  delta_stato_or_iniz : Outport  Port=2
  Outport : Outport  Port=3
  wires:
  MATLAB Function/2(delta_current_or_iniz) -> delta_current_or_iniz/1
  MATLAB Function/1(delta_stato_or_iniz) -> delta_stato_or_iniz/1
  Mux/1 -> Outport/1
  Constant/1 -> Mux/3
  Constant1/1 -> Mux/4
  Constant2/1 -> Mux/5
  Constant3/1 -> Mux/6
  Pos_s/1 -> MATLAB Function/1(Pos_s)
  Or_s/1 -> MATLAB Function/2(Or_s)
  Or_in/1 -> MATLAB Function/3(Or_in)
  MATLAB Function/3(Pos_d) -> Mux/1
  MATLAB Function/4(Or_d) -> Mux/2
  error_flag/1 -> MATLAB Function/4(error_flag)

== system sim_all/Mission_supervisor_v3/Mission_Supervisor/Orientazione in profondità ==
  Pos_s : Inport
  Orp_s : Inport  Port=2
  Punto_iniz_patt : Inport  Port=3
  error_flag : Inport  Port=4
  Action Port : ActionPort  ActionPortLabel=case [ 104 ]:
  Constant{,1..3,6} (5 alike) : Constant  Value=nan
  MATLAB Function : MATLAB Function  TreatAsAtomicUnit=on  SystemSampleTime=Ts_supervisor
  Mux : Mux  Inputs=6
  Mux1 : Mux  Inputs=3
  delta_current_or_prof : Outport
  delta_stato_or_prof : Outport  Port=2
  Outport : Outport  Port=3
  wires:
  MATLAB Function/1(delta_current_or_prof) -> delta_current_or_prof/1
  MATLAB Function/2(delta_stato_or_prof) -> delta_stato_or_prof/1
  MATLAB Function/3(Pos_d) -> Mux/1
  Mux/1 -> Outport/1
  Constant1/1 -> Mux/3
  MATLAB Function/4(Dpp_d) -> Mux/4
  MATLAB Function/5(Orp_d) -> Mux/6
  Constant/1 -> Mux1/1
  Constant2/1 -> Mux1/2
  Constant6/1 -> Mux1/3
  Mux1/1 -> Mux/2
  Constant3/1 -> Mux/5
  Pos_s/1 -> MATLAB Function/1(Pos_s)
  Orp_s/1 -> MATLAB Function/2(Orp_s)
  Punto_iniz_patt/1 -> MATLAB Function/3(punto_iniz_patt)
  error_flag/1 -> MATLAB Function/4(error_flag)

== system sim_all/Mission_supervisor_v3/Mission_Supervisor/Orientazione in superficie ==
  Or_in : Inport
  error_flag : Inport  Port=2
  punto_iniz_patt : Inport  Port=3
  Pos_s : Inport  Port=4
  Or_s : Inport  Port=5
  Action Port : ActionPort  ActionPortLabel=case [ 302 ]:
  Constant{1..2,4..5} (4 alike) : Constant  Value=nan
  MATLAB Function : MATLAB Function  TreatAsAtomicUnit=on  SystemSampleTime=Ts_supervisor
  Mux : Mux  Inputs=6
  delta_current_or_sup : Outport
  delta_stato_or_sup : Outport  Port=2
  Outport : Outport  Port=3
  wires:
  Mux/1 -> Outport/1
  Constant1/1 -> Mux/3
  Constant4/1 -> Mux/5
  Or_in/1 -> MATLAB Function/1(Or_in)
  error_flag/1 -> MATLAB Function/2(error_flag)
  punto_iniz_patt/1 -> MATLAB Function/3(punto_iniz_patt)
  MATLAB Function/1(delta_current_or_sup) -> delta_current_or_sup/1
  MATLAB Function/2(delta_stato_or_sup) -> delta_stato_or_sup/1
  MATLAB Function/4(Or_d) -> Mux/2
  MATLAB Function/3(Pos_d) -> Mux/1
  Constant2/1 -> Mux/4
  Constant5/1 -> Mux/6
  Pos_s/1 -> MATLAB Function/4(Pos_s)
  Or_s/1 -> MATLAB Function/5(Or_s)

== system sim_all/Mission_supervisor_v3/Mission_Supervisor/Pattugliamento ==
  parete : Inport
  contatore : Inport  Port=2
  Pos_s : Inport  Port=3
  Dpp_s : Inport  Port=4
  Dps_s : Inport  Port=5
  Orp_s : Inport  Port=6
  Vel_s : Inport  Port=7
  error_flag : Inport  Port=8
  giro : Inport  Port=9
  Action Port : ActionPort  ActionPortLabel=case [ 201 ]:
  Constant{,1..2,6} (4 alike) : Constant  Value=nan
  MATLAB Function : MATLAB Function  TreatAsAtomicUnit=on  SystemSampleTime=Ts_supervisor
  Mux : Mux  Inputs=6
  Mux1 : Mux  Inputs=3
  delta_current_patt : Outport
  delta_stato_patt : Outport  Port=2
  Outport : Outport  Port=3
  wires:
  MATLAB Function/1(delta_current_patt) -> delta_current_patt/1
  MATLAB Function/2(delta_stato_patt) -> delta_stato_patt/1
  parete/1 -> MATLAB Function/1(parete)
  contatore/1 -> MATLAB Function/2(contatore)
  MATLAB Function/3(Pos_d) -> Mux/1
  Mux/1 -> Outport/1
  Mux1/1 -> Mux/2
  MATLAB Function/4(Vel_d) -> Mux/3
  MATLAB Function/5(Dpp_d) -> Mux/4
  Constant/1 -> Mux1/1
  Constant2/1 -> Mux1/2
  Constant6/1 -> Mux1/3
  Pos_s/1 -> MATLAB Function/3(Pos_s)
  Dpp_s/1 -> MATLAB Function/4(Dpp_s)
  Dps_s/1 -> MATLAB Function/5(Dps_s)
  Vel_s/1 -> MATLAB Function/7(Vel_s)
  Orp_s/1 -> MATLAB Function/6(Orp_s)
  error_flag/1 -> MATLAB Function/8(error_flag)
  giro/1 -> MATLAB Function/9(giro)
  Constant1/1 -> Mux/5
  MATLAB Function/6(Orp_d) -> Mux/6

== system sim_all/Mission_supervisor_v3/Mission_Supervisor/Posizionamento ==
  Pos_s : Inport
  Or_s : Inport  Port=2
  punto iniziale : Inport  Port=3
  Or_in : Inport  Port=4
  error_flag : Inport  Port=5
  Action Port : ActionPort  ActionPortLabel=case [ 102 ]:
  Constant{,1..3} (4 alike) : Constant  Value=nan
  MATLAB Function : MATLAB Function  TreatAsAtomicUnit=on  SystemSampleTime=Ts_supervisor
  Mux : Mux  Inputs=6
  delta_current_posiz : Outport
  delta_stato_posiz : Outport  Port=2
  Outport : Outport  Port=3
  wires:
  MATLAB Function/1(delta_current_posiz) -> delta_current_posiz/1
  MATLAB Function/2(delta_stato_posiz) -> delta_stato_posiz/1
  MATLAB Function/3(Pos_d) -> Mux/1
  MATLAB Function/4(Or_d) -> Mux/2
  Mux/1 -> Outport/1
  Constant/1 -> Mux/3
  Constant1/1 -> Mux/6
  Constant2/1 -> Mux/5
  Pos_s/1 -> MATLAB Function/1(Pos_s)
  punto iniziale/1 -> MATLAB Function/3(punto_iniziale)
  Or_in/1 -> MATLAB Function/4(Or_in)
  Or_s/1 -> MATLAB Function/2(Or_s)
  error_flag/1 -> MATLAB Function/5(error_flag)
  Constant3/1 -> Mux/4

== system sim_all/Mission_supervisor_v3/Mission_Supervisor/Rientro ==
  Pos_s : Inport
  Or_in : Inport  Port=2
  error_flag : Inport  Port=3
  Dps_s : Inport  Port=4
  Dpp_s : Inport  Port=5
  Or_s : Inport  Port=6
  Action Port : ActionPort  ActionPortLabel=case [ 303 ]:
  Constant{1..4} (4 alike) : Constant  Value=nan
  MATLAB Function : MATLAB Function  TreatAsAtomicUnit=on  SystemSampleTime=Ts_supervisor
  Mux : Mux  Inputs=6
  delta_current_rient : Outport
  delta_stato_rient : Outport  Port=2
  Outport : Outport  Port=3
  wires:
  MATLAB Function/1(delta_current_rient) -> delta_current_rient/1
  MATLAB Function/2(delta_stato_rient) -> delta_stato_rient/1
  MATLAB Function/3(Pos_d) -> Mux/1
  Mux/1 -> Outport/1
  Constant1/1 -> Mux/3
  Constant2/1 -> Mux/4
  Constant3/1 -> Mux/5
  Constant4/1 -> Mux/6
  Pos_s/1 -> MATLAB Function/1(Pos_s)
  MATLAB Function/4(Or_d) -> Mux/2
  Or_in/1 -> MATLAB Function/2(Or_in)
  error_flag/1 -> MATLAB Function/3(error_flag)
  Dps_s/1 -> MATLAB Function/4(Dps_s)
  Dpp_s/1 -> MATLAB Function/5(Dpp_s)
  Or_s/1 -> MATLAB Function/6(Or_s)

== system sim_all/Mission_supervisor_v3/Mission_Supervisor/Risalita ==
  delta_SOS : Inport
  Pos_s : Inport  Port=2
  Dpp_s : Inport  Port=3
  Orp_s : Inport  Port=4
  Dps_s : Inport  Port=5
  Dps_fin : Inport  Port=6
  error_flag : Inport  Port=7
  SOS_205 : Inport  Port=8
  Action Port : ActionPort  ActionPortLabel=case [ 301 ]:
  Constant{,1,3,6} (4 alike) : Constant  Value=nan
  MATLAB Function : MATLAB Function  TreatAsAtomicUnit=on  SystemSampleTime=Ts_supervisor
  Mux : Mux  Inputs=6
  Mux1 : Mux  Inputs=3
  delta_current_ris : Outport
  delta_stato_ris : Outport  Port=2
  Outport : Outport  Port=3
  wires:
  MATLAB Function/1(delta_current_ris) -> delta_current_ris/1
  MATLAB Function/2(delta_stato_ris) -> delta_stato_ris/1
  MATLAB Function/3(Pos_d) -> Mux/1
  Mux/1 -> Outport/1
  Mux1/1 -> Mux/2
  Constant1/1 -> Mux/3
  MATLAB Function/4(Dpp_d) -> Mux/4
  Constant/1 -> Mux1/1
  Constant3/1 -> Mux1/2
  Constant6/1 -> Mux1/3
  MATLAB Function/5(Dps_d) -> Mux/5
  Pos_s/1 -> MATLAB Function/2(Pos_s)
  Dpp_s/1 -> MATLAB Function/3(Dpp_s)
  MATLAB Function/6(Orp_d) -> Mux/6
  delta_SOS/1 -> MATLAB Function/1(delta_SOS)
  Orp_s/1 -> MATLAB Function/4(Orp_s)
  Dps_s/1 -> MATLAB Function/5(Dps_s)
  Dps_fin/1 -> MATLAB Function/6(Dps_fin)
  error_flag/1 -> MATLAB Function/7(error_flag)
  SOS_205/1 -> MATLAB Function/8(SOS_205)

== system sim_all/Model/Vehicle Model/P1 ==
  note: n is the rotational speed of the thruster
      | V is the speed component of the water along the thruster axis
      |
      | n is saturated according to data
      | a dead zone is considered according to data
      | the thruster is characterised by 1st order dynamics (tau = 0.2s)
  n1 [rad/s] : Inport
  V1 [m/s] : Inport  Port=2
  Dead Zone : DeadZone  LowerValue=-dead_zone_limit  UpperValue=dead_zone_limit  SaturateOnIntegerOverflow=on
  Propeller1 : MATLAB Function  TreatAsAtomicUnit=on
  Saturation : Saturate  UpperLimit=n_max  LowerLimit=-n_max
  Transfer Fcn : TransferFcn  Denominator=[0.2 1]
  T1 : Outport
  wires:
  V1 [m/s]/1 -> Propeller1/2(V1)
  Saturation/1 -> Propeller1/1(n1)
  Transfer Fcn/1 -> Saturation/1
  Dead Zone/1 -> Transfer Fcn/1
  n1 [rad/s]/1 -> Dead Zone/1
  Propeller1/1(T1) -> T1/1

== system sim_all/Model/Vehicle Model/P2 ==
  note: n is the rotational speed of the thruster
      | V is the speed component of the water along the thruster axis
      |
      | n is saturated according to data
      | a dead zone is considered according to data
      | the thruster is characterised by 1st order dynamics (tau = 0.2s)
  n2 [rad/s] : Inport
  V2 [m/s] : Inport  Port=2
  Dead Zone : DeadZone  LowerValue=-dead_zone_limit  UpperValue=dead_zone_limit  SaturateOnIntegerOverflow=on
  Propeller2 : MATLAB Function  TreatAsAtomicUnit=on
  Saturation : Saturate  UpperLimit=n_max  LowerLimit=-n_max
  Transfer Fcn : TransferFcn  Denominator=[0.2 1]
  T2 : Outport
  wires:
  V2 [m/s]/1 -> Propeller2/2(V2)
  Saturation/1 -> Propeller2/1(n2)
  Transfer Fcn/1 -> Saturation/1
  Dead Zone/1 -> Transfer Fcn/1
  n2 [rad/s]/1 -> Dead Zone/1
  Propeller2/1(T2) -> T2/1
